simulink model "p2"  (R2015a)
settings: Solver=ode45  StartTime=0.0  StopTime=10.0  RelTol=1e-3
values from neighbouring files (symbols this model uses):
  g = 9.81    [env.m]
  l = 10    [env.m]
  x0 = [pi/2 0]    [env.m]
libraries: simulink x1
settings Model: Creator=jgutierr  LastModifiedBy=vdrouinv

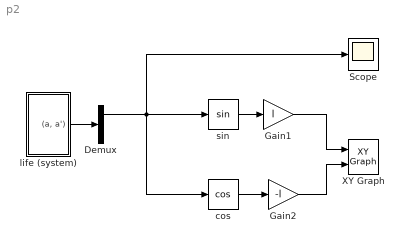
== system p2 ==
  Demux : Demux  Outputs=2
  Gain1 : Gain  Gain=l
  Gain2 : Gain  Gain=-l
  Scope : Scope
  XY Graph : simulink/Sinks/XY Graph  xmin=-10  xmax=10  ymin=-10  ymax=10  st=-1
  cos : Trigonometry  Operator=cos
  life (system) : Subsystem
  sin : Trigonometry
  wires:
  Gain1/1 -> XY Graph/1
  Gain2/1 -> XY Graph/2
  cos/1 -> Gain2/1
  sin/1 -> Gain1/1
  Demux/1 -> Scope/1, sin/1, cos/1
  life (system)/1("(a, a')") -> Demux/1

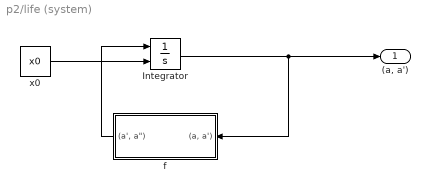
== system p2/life (system) ==
  Integrator : Integrator  InitialConditionSource=external
  f : Subsystem
  x0 : Constant  Value=x0
  "(a, a')" : Outport
  wires:
  x0/1 -> Integrator/2
  f/1("(a', a\")") -> Integrator/1
  Integrator/1 -> "(a, a')"/1, f/1("(a, a')")

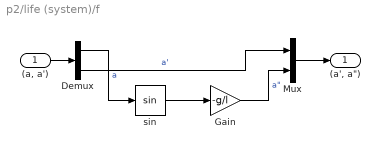
== system p2/life (system)/f ==
  "(a, a')" : Inport
  Demux : Demux  Outputs=2
  Gain : Gain  Gain=-g/l
  Mux : Mux  Inputs=2
  sin : Trigonometry
  "(a', a\")" : Outport
  wires:
  Gain/1 -> Mux/2  "a\""
  Demux/1 -> sin/1  "a"
  Demux/2 -> Mux/1  "a'"
  sin/1 -> Gain/1
  "(a, a')"/1 -> Demux/1
  Mux/1 -> "(a', a\")"/1
